simulink model "example1_3"  (R2016b)
settings: Solver=VariableStepAuto  StartTime=0.0  StopTime=5  RelTol=1e-3
values from neighbouring files (symbols this model uses):
  A = [0 1 0 0;-4 -2 4 2;0 0 0 1;2 1 -2 -1]    [example1_3.m]
  B = [0;1;0;0]    [example1_3.m]
  C = [0,0,1,0]    [example1_3.m]
  h = 7.75    [example1_3.m]
  k = [-1.9, -1.71, -5.84, -4.45]    [example1_3.m]
settings Model: Creator=Trancemania  LastModifiedBy=Trancemania

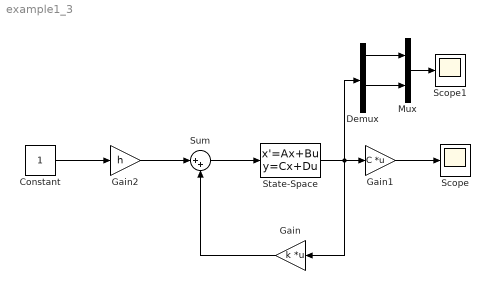
== system example1_3 ==
  Constant : Constant
  Demux : Demux
  Gain : Gain  Gain=k  Multiplication=Matrix(K*u)
  Gain1 : Gain  Gain=C  Multiplication=Matrix(K*u)
  Gain2 : Gain  Gain=h
  Mux : Mux  Inputs=2
  Scope : Scope
  Scope1 : Scope
  State-Space : StateSpace  A=A  B=B  C=eye(4)  D=zeros(4,1)  X0=0
  Sum : Sum  Inputs=|++
  wires:
  State-Space/1 -> Demux/1, Gain/1, Gain1/1
  Sum/1 -> State-Space/1
  Gain/1 -> Sum/2
  Gain2/1 -> Sum/1
  Constant/1 -> Gain2/1
  Gain1/1 -> Scope/1
  Demux/1 -> Mux/1
  Demux/3 -> Mux/2
  Mux/1 -> Scope1/1
